simulink model "cx06_MA"  (Simulink 7.5)
settings: Solver=FixedStepDiscrete  StartTime=0.0  StopTime=10.0  RelTol=1e-3
undefined symbols (not defined in the file or in its folder): DiscIntNeverNeededParam, ECU555, int, motohawk_build_version, motohawk_trunc_name, motohawk_vardec_path
libraries: MotoHawk_lib x811, simulink x43, simulink_need_slupdate x1
(part 4 of 10)

== system cx06_MA/Outputs/Drive-by-Wire CAN Output ==
  Outputs : Inport  OutDataType=sfix(16)  OutScaling=2^0
  Bus Selector : BusSelector  OutputSignals=Hybrid.engine_Torque
  Constant : Constant  Value=0  OutDataType=sfix(16)  OutScaling=2^0
  Constant1 : Constant  Value=0  OutDataType=sfix(16)  OutScaling=2^0
  Data Type Conversion{,1..3} (4 alike) : DataTypeConversion  OutDataTypeMode=uint16  OutDataType=sfix(16)  OutScaling=2^0  OutDataTypeStr=uint16
  Gain1 : Gain  Gain=hex2dec('FFF')/5  ParameterDataType=sfix(16)  ParameterScaling=2^0  OutDataTypeMode=Specify via dialog  OutDataType=sint(16)  OutDataTypeStr=sint(16)
  Gain2 : Gain  Gain=hex2dec('FFF')/5  ParameterDataType=sfix(16)  ParameterScaling=2^0  OutDataTypeMode=Specify via dialog  OutDataType=sint(16)  OutDataTypeStr=sint(16)
  Product : Product  OutDataType=sfix(16)  OutScaling=2^0  RndMeth=Zero
  Product1 : Product  OutDataType=sfix(16)  OutScaling=2^0  RndMeth=Zero
  Send CAN Messages : MotoHawk_lib/CAN Blocks/Send CAN Messages  bus=-2  nam=['CAN_' num2str(1)]  msgl=CANTx_AO_169  pace=5  labelwires=on
  Subsystem : Subsystem
  Sum : Sum  Inputs=-+  OutDataType=sfix(16)  OutScaling=2^0
  Sum1 : Sum  Inputs=++|  OutDataType=sfix(16)  OutScaling=2^0
  Sum2 : Sum  Inputs=-+  OutDataType=sfix(16)  OutScaling=2^0
  Sum3 : Sum  Inputs=++|  OutDataType=sfix(16)  OutScaling=2^0
  motohawk_calibration : MotoHawk_lib/Calibration & Probing Blocks/motohawk_calibration  nam='Out1_Zero'  val=1  storage=Calibration  show_more=on  name_source=Use Parameter  data_type=Inherit from 'Default Value'  read_level=1  write_level=1  ovr_cals=on  view_as=Number  enum_struct={'Disabled', 'Enabled'}  vector_style=Wide Row  use_help_units=on  help='Output 0% Voltage'  units='V'  use_header_enum=off  row_header_enum={}  col_header_enum={}  use_min_max=off  min_val=0  max_val=5  use_precision=on  precision='1.3'  gain=1  offset=0  exp=1  use_mototune_group=off  mototune_group=motohawk_vardec_path(gcb)
  motohawk_calibration1 : MotoHawk_lib/Calibration & Probing Blocks/motohawk_calibration  nam='Out1_Full'  val=3.55  storage=Calibration  show_more=on  name_source=Use Parameter  data_type=Inherit from 'Default Value'  read_level=1  write_level=1  ovr_cals=on  view_as=Number  enum_struct={'Disabled', 'Enabled'}  vector_style=Wide Row  use_help_units=on  help='Output 100% Voltage'  units='V'  use_header_enum=off  row_header_enum={}  col_header_enum={}  use_min_max=off  min_val=0  max_val=5  use_precision=on  precision='1.3'  gain=1  offset=0  exp=1  use_mototune_group=off  mototune_group=motohawk_vardec_path(gcb)
  motohawk_calibration2 : MotoHawk_lib/Calibration & Probing Blocks/motohawk_calibration  nam='Out2_Zero'  val=0.5  storage=Calibration  show_more=on  name_source=Use Parameter  data_type=Inherit from 'Default Value'  read_level=1  write_level=1  ovr_cals=on  view_as=Number  enum_struct={'Disabled', 'Enabled'}  vector_style=Wide Row  use_help_units=on  help='Output1 0 Voltage'  units='V'  use_header_enum=off  row_header_enum={}  col_header_enum={}  use_min_max=off  min_val=0  max_val=5  use_precision=on  precision='1.3'  gain=1  offset=0  exp=1  use_mototune_group=off  mototune_group=motohawk_vardec_path(gcb)
  motohawk_calibration3 : MotoHawk_lib/Calibration & Probing Blocks/motohawk_calibration  nam='Out2_Full'  val=1.750  storage=Calibration  show_more=on  name_source=Use Parameter  data_type=Inherit from 'Default Value'  read_level=1  write_level=1  ovr_cals=on  view_as=Number  enum_struct={'Disabled', 'Enabled'}  vector_style=Wide Row  use_help_units=on  help='Output 100% Voltage'  units='V'  use_header_enum=off  row_header_enum={}  col_header_enum={}  use_min_max=off  min_val=0  max_val=5  use_precision=on  precision='1.3'  gain=1  offset=0  exp=1  use_mototune_group=off  mototune_group=motohawk_vardec_path(gcb)
  motohawk_override_abs{,1..3} (4 alike) : MotoHawk_lib/Calibration & Probing Blocks/motohawk_override_abs  SystemSampleTime=-1  parent_name='Override_Absolute'  parent_val=0  show_more=on  name_source=Use Output Wire Name  parent_read_level=1  parent_override_level=1  view_as=Number  enum_struct={'Disabled', 'Enabled'}  use_help_units=off  parent_help=''  parent_units=''  use_min_max=off  parent_min=-inf  parent_max=inf  use_precision=off  parent_precision=''  parent_gain=1  parent_offset=0  parent_exp=1  use_mototune_group=off  parent_group=motohawk_vardec_path(gcb)
  motohawk_probe{,1..3} (4 alike) : MotoHawk_lib/Calibration & Probing Blocks/motohawk_probe  nam='Probe'  show_more=on  name_source=Use Input Wire Name  read_level=1  view_as=Number  enum_struct={'Disabled', 'Enabled'}  vector_style=Wide Row  use_help_units=off  help=''  units=''  use_header_enum=off  row_header_enum={}  col_header_enum={}  use_precision=off  precision=''  gain=1  offset=0  exp=1  use_mototune_group=off  mototune_group=motohawk_vardec_path(gcb)
  motohawk_probe4 : MotoHawk_lib/Calibration & Probing Blocks/motohawk_probe  nam='AO_Checksum'  show_more=on  name_source=Use Parameter  read_level=1  view_as=Number  enum_struct={'Disabled', 'Enabled'}  vector_style=Wide Row  use_help_units=off  help=''  units=''  use_header_enum=off  row_header_enum={}  col_header_enum={}  use_precision=off  precision=''  gain=1  offset=0  exp=1  use_mototune_group=off  mototune_group=motohawk_vardec_path(gcb)
  wires:
  motohawk_override_abs/1 -> motohawk_probe1/1, Data Type Conversion2/1  "Reset_AO1"
  motohawk_override_abs1/1 -> motohawk_probe/1, Gain2/1  "Output_1"
  motohawk_override_abs2/1 -> motohawk_probe2/1, Data Type Conversion3/1  "Reset_AO2"
  motohawk_override_abs3/1 -> motohawk_probe3/1, Gain1/1  "Output_2"
  Constant/1 -> motohawk_override_abs/1  "Reset_AO1"
  Constant1/1 -> motohawk_override_abs2/1  "Reset_AO2"
  Sum/1 -> Product/1
  motohawk_calibration/1 -> Sum/1, Sum1/1
  motohawk_calibration1/1 -> Sum/2
  Product/1 -> Sum1/2
  Sum1/1 -> motohawk_override_abs1/1  "Output_1"
  Sum2/1 -> Product1/1
  motohawk_calibration2/1 -> Sum3/1, Sum2/1
  motohawk_calibration3/1 -> Sum2/2
  Product1/1 -> Sum3/2
  Sum3/1 -> motohawk_override_abs3/1  "Output_2"
  Outputs/1 -> Bus Selector/1
  Bus Selector/1 -> Product/2, Product1/2  "<engine_Torque>"
  Subsystem/1(Checksum) -> Send CAN Messages/5, motohawk_probe4/1  "Parity"
  Gain1/1 -> Data Type Conversion1/1  "Output_2"
  Gain2/1 -> Data Type Conversion/1  "Output_1"
  Data Type Conversion/1 -> Send CAN Messages/2, Subsystem/2(Output1)  "Output_1"
  Data Type Conversion1/1 -> Send CAN Messages/4, Subsystem/4(Output2)  "Output_2"
  Data Type Conversion2/1 -> Send CAN Messages/1, Subsystem/1(Reset_AO1)  "Reset_AO1"
  Data Type Conversion3/1 -> Send CAN Messages/3, Subsystem/3(Reset_AO2)  "Reset_AO2"

== system cx06_MA/Outputs/Fiat CAN Output ==
  note: NOTE:
      | Message $2F0
      | allows ECU to do
      | "supervisory checking"
      | on ABS
  Inputs : Inport  OutDataType=sfix(16)  OutScaling=2^0
  Bus Selector1 : BusSelector  OutputSignals=GMLAN.FL_Whl_Spd,GMLAN.FR_Whl_Spd,GMLAN.RL_Whl_Spd,GMLAN.RR_Whl_Spd
  Constant : Constant  OutDataType=sfix(16)  OutScaling=2^0
  Constant1 : Constant  Value=0  OutDataType=sfix(16)  OutScaling=2^0
  MinMax{,1..3} (4 alike) : MinMax  Function=max  Inputs=2  OutDataType=sfix(16)  OutScaling=2^0
  Send CAN Messages : MotoHawk_lib/CAN Blocks/Send CAN Messages  bus=-2  nam=['CAN_' num2str(1)]  msgl=CANTx_FIAT_280  pace=2  labelwires=on
  Send CAN Messages1 : MotoHawk_lib/CAN Blocks/Send CAN Messages  bus=-2  nam=['CAN_' num2str(1)]  msgl=CANTx_FIAT_2F0  pace=2  labelwires=on
  motohawk_calibration : MotoHawk_lib/Calibration & Probing Blocks/motohawk_calibration  nam='Wheel_Speed_Validities'  val=0  storage=Calibration  show_more=on  name_source=Use Parameter  data_type=uint8  read_level=1  write_level=1  ovr_cals=on  view_as=Enumeration  enum_struct={'Valid', 'Invalid'}  vector_style=Wide Row  use_help_units=on  help='Sets Validity bit for each wheels output on CAN'  units=''  use_header_enum=off  row_header_enum={}  col_header_enum={}  use_min_max=off  min_val=-inf  max_val=inf  use_precision=off  precision=''  gain=1  offset=0  exp=1  use_mototune_group=off  mototune_group=motohawk_vardec_path(gcb)
  motohawk_calibration1 : MotoHawk_lib/Calibration & Probing Blocks/motohawk_calibration  nam='Min_Wheel_Vel'  val=0  storage=Calibration  show_more=on  name_source=Use Parameter  data_type=double  read_level=1  write_level=1  ovr_cals=on  view_as=Number  enum_struct={'Valid', 'Invalid'}  vector_style=Wide Row  use_help_units=on  help='prevents ECU derating in first gear'  units=''  use_header_enum=off  row_header_enum={}  col_header_enum={}  use_min_max=off  min_val=-inf  max_val=inf  use_precision=on  precision='3.1'  gain=1  offset=0  exp=1  use_mototune_group=off  mototune_group=motohawk_vardec_path(gcb)
  motohawk_override_abs{,1..7} (8 alike) : MotoHawk_lib/Calibration & Probing Blocks/motohawk_override_abs  SystemSampleTime=-1  parent_name='Override_Absolute'  parent_val=0  show_more=on  name_source=Use Output Wire Name  parent_read_level=1  parent_override_level=1  view_as=Number  enum_struct={'Disabled', 'Enabled'}  use_help_units=off  parent_help=''  parent_units=''  use_min_max=off  parent_min=-inf  parent_max=inf  use_precision=off  parent_precision=''  parent_gain=1  parent_offset=0  parent_exp=1  use_mototune_group=off  parent_group=motohawk_vardec_path(gcb)
  motohawk_probe{,1..7} (8 alike) : MotoHawk_lib/Calibration & Probing Blocks/motohawk_probe  nam='Probe'  show_more=on  name_source=Use Input Wire Name  read_level=1  view_as=Number  enum_struct={'Disabled', 'Enabled'}  vector_style=Wide Row  use_help_units=off  help=''  units=''  use_header_enum=off  row_header_enum={}  col_header_enum={}  use_precision=off  precision=''  gain=1  offset=0  exp=1  use_mototune_group=off  mototune_group=motohawk_vardec_path(gcb)
  wires:
  Inputs/1 -> Bus Selector1/1
  motohawk_override_abs/1 -> Send CAN Messages/1, motohawk_probe/1  "Wheel_Ang_Vel_FL_V"
  motohawk_override_abs1/1 -> Send CAN Messages/2, motohawk_probe1/1  "Wheel_Ang_Vel_FL"
  motohawk_override_abs2/1 -> Send CAN Messages/3, motohawk_probe2/1  "Wheel_Ang_Vel_FR_V"
  motohawk_override_abs3/1 -> Send CAN Messages/4, motohawk_probe3/1  "Wheel_Ang_Vel_FR"
  motohawk_override_abs4/1 -> Send CAN Messages/5, motohawk_probe4/1  "Wheel_Ang_Vel_RL_V"
  motohawk_override_abs5/1 -> Send CAN Messages/6, motohawk_probe5/1  "Wheel_Ang_Vel_RL"
  motohawk_override_abs6/1 -> Send CAN Messages/7, motohawk_probe6/1  "Wheel_Ang_Vel_RR_V"
  motohawk_override_abs7/1 -> Send CAN Messages/8, motohawk_probe7/1  "Wheel_Ang_Vel_RR"
  motohawk_calibration/1 -> motohawk_override_abs/1, motohawk_override_abs2/1, motohawk_override_abs4/1, motohawk_override_abs6/1  "Wheel_Ang_Vel_RR_V"
  Constant1/1 -> Send CAN Messages1/1, Send CAN Messages1/4, Send CAN Messages1/5, Send CAN Messages1/6, Send CAN Messages1/7, Send CAN Messages1/8, Send CAN Messages1/9, Send CAN Messages1/11, Send CAN Messages1/12, Send CAN Messages1/19, Send CAN Messages1/20, Send CAN Messages1/21, Send CAN Messages1/23, Send CAN Messages1/24, Send CAN Messages1/26, Send CAN Messages1/25, Send CAN Messages1/18, Send CAN Messages1/17, Send CAN Messages1/16, Send CAN Messages1/15, Send CAN Messages1/14, Send CAN Messages1/13, Send CAN Messages1/10  "Drv_Off_Assist_Status"
  Constant/1 -> Send CAN Messages1/2, Send CAN Messages1/3, Send CAN Messages1/22  "Brk_Pres_Sensor_Diag_Complete"
  MinMax/1 -> motohawk_override_abs1/1  "Wheel_Ang_Vel_FL"
  Bus Selector1/1 -> MinMax/1  "<FL_Whl_Spd>"
  MinMax1/1 -> motohawk_override_abs3/1  "Wheel_Ang_Vel_FR"
  Bus Selector1/2 -> MinMax1/1  "<FR_Whl_Spd>"
  motohawk_calibration1/1 -> MinMax1/2, MinMax/2, MinMax2/2, MinMax3/2
  MinMax2/1 -> motohawk_override_abs5/1  "Wheel_Ang_Vel_RL"
  Bus Selector1/3 -> MinMax2/1  "<RL_Whl_Spd>"
  Bus Selector1/4 -> MinMax3/1  "<RR_Whl_Spd>"
  MinMax3/1 -> motohawk_override_abs7/1  "Wheel_Ang_Vel_RR"

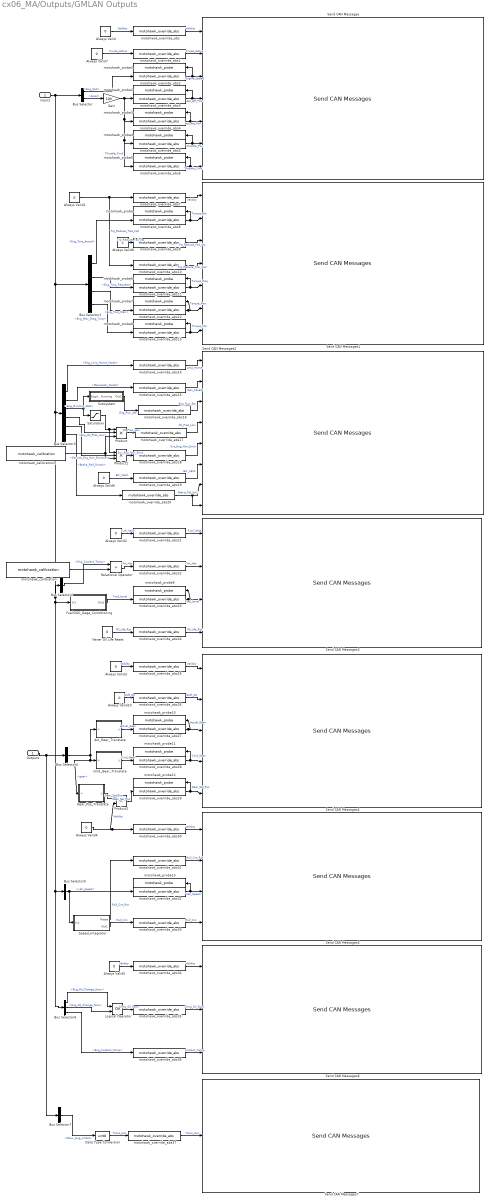
== system cx06_MA/Outputs/GMLAN Outputs ==
  Outputs : Inport  OutDataType=sfix(16)  OutScaling=2^0
  Inputs : Inport  Port=2  OutDataType=sfix(16)  OutScaling=2^0
  Act_Gear_Translate : Stateflow chart  TreatAsAtomicUnit=on
  Always Valid{,1..7,10} (9 alike) : Constant  Value=0  OutDataType=sfix(16)  OutScaling=2^0
  Always Valid8 : Constant  Value=2  OutDataType=sfix(16)  OutScaling=2^0
  Bus Selector : BusSelector  OutputSignals=Fiat.Engine Speed and Pedal Pos.Eng_Spd,Analog.Driver.Accel
  Bus Selector1 : BusSelector  OutputSignals=Fiat.Engine Torque.Eng_Torq_Actual,Fiat.Engine Torque.Eng_Torq_Request,Fiat.Engine Torque.Eng_Torq_Max,Fiat.Engine Torque.Eng_Max_Drag_Torq
  Bus Selector2 : BusSelector  OutputSignals=Fiat.Engine Temp.Eng_Coolant_Temp
  Bus Selector3 : BusSelector  OutputSignals="Fiat.Engine  General Status.Eng_Limp_Home_Mode,Fiat.Engine  General Status.Generator_Failed,Fiat.Engine  General Status.Eng_Running_Stat,Fiat.Engine  General Status.Eng_Oil_Pres_Low,Fiat.Engine  General Status.Service_Eng_Non_Emission,Fiat.Engine  General Status.Brake_Ped_Switch"
  Bus Selector4 : BusSelector  OutputSignals=Fiat/GMLAN.gear
  Bus Selector5 : BusSelector  OutputSignals=IPT.Status 2.veh_speed
  Bus Selector6 : BusSelector  OutputSignals="Fiat.Engine  General Status.Eng_Oil_Change_Soon,Fiat.Engine  General Status.Eng_Oil_Change_Now,Fiat.Engine Temp.Eng_Coolant_Temp"
  Bus Selector7 : BusSelector  OutputSignals=Hybrid.ESS_Outputs.Glow_plug_inhibit
  Cmd_Gear_Translate : Stateflow chart  TreatAsAtomicUnit=on
  Data Type Conversion : DataTypeConversion  OutDataTypeMode=uint8  OutDataType=sfix(16)  OutScaling=2^0  OutDataTypeStr=uint8
  Fuel/SOC_Gage_Conditioning : Subsystem
  Gain : Gain  Gain=100  ParameterDataType=sfix(16)  ParameterScaling=2^0  OutDataType=sfix(16)  OutScaling=2^0
  Gear_Pos_Translate : Stateflow chart  TreatAsAtomicUnit=on
  Logical Operator : Logic  Operator=OR  AllPortsSameDT=off  OutDataTypeMode=boolean  OutDataTypeStr=boolean
  Never Oil Life Reset : Constant  Value=0  OutDataType=sfix(16)  OutScaling=2^0
  Product : Product  Inputs=3  OutDataType=sfix(16)  OutScaling=2^0  RndMeth=Zero
  Product1 : Product  Inputs=3  OutDataType=sfix(16)  OutScaling=2^0  RndMeth=Zero
  Product2 : Product  OutDataType=sfix(16)  OutScaling=2^0  RndMeth=Zero
  Relational Operator : RelationalOperator  Operator=>  LogicOutDataTypeMode=boolean  OutDataTypeStr=boolean
  Saturation : Saturate  UpperLimit=1  LowerLimit=0
  Send CAN Messages : MotoHawk_lib/CAN Blocks/Send CAN Messages  bus=-2  nam=['CAN_' num2str(2)]  msgl=CANTx_GMLAN_110  pace=5  labelwires=on
  Send CAN Messages1 : MotoHawk_lib/CAN Blocks/Send CAN Messages  bus=-2  nam=['CAN_' num2str(2)]  msgl=CANTx_GMLAN_120  pace=5  labelwires=on
  Send CAN Messages2 : MotoHawk_lib/CAN Blocks/Send CAN Messages  bus=-2  nam=['CAN_' num2str(2)]  msgl=CANTx_GMLAN_300  pace=5  labelwires=on
  Send CAN Messages3 : MotoHawk_lib/CAN Blocks/Send CAN Messages  bus=-2  nam=['CAN_' num2str(2)]  msgl=CANTx_GMLAN_308  pace=5  labelwires=on
  Send CAN Messages4 : MotoHawk_lib/CAN Blocks/Send CAN Messages  bus=-2  nam=['CAN_' num2str(2)]  msgl=CANTx_GMLAN_320  pace=5  labelwires=on
  Send CAN Messages5 : MotoHawk_lib/CAN Blocks/Send CAN Messages  bus=-2  nam=['CAN_' num2str(2)]  msgl=CANTx_GMLAN_410  pace=5  labelwires=on
  Send CAN Messages6 : MotoHawk_lib/CAN Blocks/Send CAN Messages  bus=-2  nam=['CAN_' num2str(2)]  msgl=CANTx_GMLAN_510  pace=5  labelwires=on
  Send CAN Messages7 : MotoHawk_lib/CAN Blocks/Send CAN Messages  bus=-2  nam='CAN_2'  msgl=CANTx_GMLAN_520  pace=5  labelwires=on
  Speed_Integrator : Subsystem
  Subsystem : Subsystem
  motohawk_calibration : MotoHawk_lib/Calibration & Probing Blocks/motohawk_calibration  nam='Coolant_Temp_Warning_Thres'  val=115  storage=Calibration  show_more=off  name_source=Use Parameter  data_type=Inherit from 'Default Value'  read_level=1  write_level=1  ovr_cals=on  view_as=Number  enum_struct={'Disabled', 'Enabled'}  vector_style=Wide Row  use_help_units=off  help=''  units=''  use_header_enum=off  row_header_enum={}  col_header_enum={}  use_min_max=off  min_val=-inf  max_val=inf  use_precision=off  precision=''  gain=1  offset=0  exp=1  use_mototune_group=off  mototune_group=motohawk_vardec_path(gcb)
  motohawk_calibration1 : MotoHawk_lib/Calibration & Probing Blocks/motohawk_calibration  nam='CheckEngineLights'  val=1  storage=Calibration  show_more=on  name_source=Use Parameter  data_type=uint8  read_level=1  write_level=1  ovr_cals=on  view_as=Enumeration  enum_struct={'Disabled', 'Enabled'}  vector_style=Wide Row  use_help_units=off  help=''  units=''  use_header_enum=off  row_header_enum={}  col_header_enum={}  use_min_max=off  min_val=-inf  max_val=inf  use_precision=off  precision=''  gain=1  offset=0  exp=1  use_mototune_group=off  mototune_group=motohawk_vardec_path(gcb)
  motohawk_override_abs : MotoHawk_lib/Calibration & Probing Blocks/motohawk_override_abs  SystemSampleTime=-1  parent_name='Validity_110'  parent_val=0  show_more=on  name_source=Use Parameter  parent_read_level=1  parent_override_level=1  view_as=Number  enum_struct={'Disabled', 'Enabled'}  use_help_units=off  parent_help=''  parent_units=''  use_min_max=off  parent_min=-inf  parent_max=inf  use_precision=off  parent_precision=''  parent_gain=1  parent_offset=0  parent_exp=1  use_mototune_group=off  parent_group=motohawk_vardec_path(gcb)
  motohawk_override_abs{1..6,8..18,20,22..24,26..29,31..33,35..37} (31 alike) : MotoHawk_lib/Calibration & Probing Blocks/motohawk_override_abs  SystemSampleTime=-1  parent_name='Override_Absolute'  parent_val=0  show_more=on  name_source=Use Output Wire Name  parent_read_level=1  parent_override_level=1  view_as=Number  enum_struct={'Disabled', 'Enabled'}  use_help_units=off  parent_help=''  parent_units=''  use_min_max=off  parent_min=-inf  parent_max=inf  use_precision=off  parent_precision=''  parent_gain=1  parent_offset=0  parent_exp=1  use_mototune_group=off  parent_group=motohawk_vardec_path(gcb)
  motohawk_override_abs19 : MotoHawk_lib/Calibration & Probing Blocks/motohawk_override_abs  SystemSampleTime=-1  parent_name='Validity_300'  parent_val=0  show_more=on  name_source=Use Parameter  parent_read_level=1  parent_override_level=1  view_as=Number  enum_struct={'Disabled', 'Enabled'}  use_help_units=off  parent_help=''  parent_units=''  use_min_max=off  parent_min=-inf  parent_max=inf  use_precision=off  parent_precision=''  parent_gain=1  parent_offset=0  parent_exp=1  use_mototune_group=off  parent_group=motohawk_vardec_path(gcb)
  motohawk_override_abs21 : MotoHawk_lib/Calibration & Probing Blocks/motohawk_override_abs  SystemSampleTime=-1  parent_name='Validity_308'  parent_val=0  show_more=on  name_source=Use Parameter  parent_read_level=1  parent_override_level=1  view_as=Number  enum_struct={'Disabled', 'Enabled'}  use_help_units=off  parent_help=''  parent_units=''  use_min_max=off  parent_min=-inf  parent_max=inf  use_precision=off  parent_precision=''  parent_gain=1  parent_offset=0  parent_exp=1  use_mototune_group=off  parent_group=motohawk_vardec_path(gcb)
  motohawk_override_abs25 : MotoHawk_lib/Calibration & Probing Blocks/motohawk_override_abs  SystemSampleTime=-1  parent_name='Validity_320'  parent_val=0  show_more=on  name_source=Use Parameter  parent_read_level=1  parent_override_level=1  view_as=Number  enum_struct={'Disabled', 'Enabled'}  use_help_units=off  parent_help=''  parent_units=''  use_min_max=off  parent_min=-inf  parent_max=inf  use_precision=off  parent_precision=''  parent_gain=1  parent_offset=0  parent_exp=1  use_mototune_group=off  parent_group=motohawk_vardec_path(gcb)
  motohawk_override_abs30 : MotoHawk_lib/Calibration & Probing Blocks/motohawk_override_abs  SystemSampleTime=-1  parent_name='Validity_410'  parent_val=0  show_more=on  name_source=Use Parameter  parent_read_level=1  parent_override_level=1  view_as=Number  enum_struct={'Disabled', 'Enabled'}  use_help_units=off  parent_help=''  parent_units=''  use_min_max=off  parent_min=-inf  parent_max=inf  use_precision=off  parent_precision=''  parent_gain=1  parent_offset=0  parent_exp=1  use_mototune_group=off  parent_group=motohawk_vardec_path(gcb)
  motohawk_override_abs34 : MotoHawk_lib/Calibration & Probing Blocks/motohawk_override_abs  SystemSampleTime=-1  parent_name='Validity_510'  parent_val=0  show_more=on  name_source=Use Parameter  parent_read_level=1  parent_override_level=1  view_as=Number  enum_struct={'Disabled', 'Enabled'}  use_help_units=off  parent_help=''  parent_units=''  use_min_max=off  parent_min=-inf  parent_max=inf  use_precision=off  parent_precision=''  parent_gain=1  parent_offset=0  parent_exp=1  use_mototune_group=off  parent_group=motohawk_vardec_path(gcb)
  motohawk_override_abs7 : MotoHawk_lib/Calibration & Probing Blocks/motohawk_override_abs  SystemSampleTime=-1  parent_name='Validity_120'  parent_val=0  show_more=on  name_source=Use Parameter  parent_read_level=1  parent_override_level=1  view_as=Number  enum_struct={'Disabled', 'Enabled'}  use_help_units=off  parent_help=''  parent_units=''  use_min_max=off  parent_min=-inf  parent_max=inf  use_precision=off  parent_precision=''  parent_gain=1  parent_offset=0  parent_exp=1  use_mototune_group=off  parent_group=motohawk_vardec_path(gcb)
  motohawk_probe{,1..13} (14 alike) : MotoHawk_lib/Calibration & Probing Blocks/motohawk_probe  nam='Probe'  show_more=on  name_source=Use Input Wire Name  read_level=1  view_as=Number  enum_struct={'Disabled', 'Enabled'}  vector_style=Wide Row  use_help_units=off  help=''  units=''  use_header_enum=off  row_header_enum={}  col_header_enum={}  use_precision=off  precision=''  gain=1  offset=0  exp=1  use_mototune_group=off  mototune_group=motohawk_vardec_path(gcb)
  wires:
  motohawk_override_abs/1 -> Send CAN Messages/1  "Validity"
  motohawk_override_abs1/1 -> Send CAN Messages/2  "Cruise_Active"
  motohawk_override_abs2/1 -> Send CAN Messages/3, motohawk_probe1/1  "Engine_Speed"
  motohawk_override_abs3/1 -> Send CAN Messages/4, motohawk_probe2/1  "Acc_Eff_Pos"
  motohawk_override_abs4/1 -> Send CAN Messages/5, motohawk_probe3/1  "Acc_Act_Pos"
  motohawk_override_abs5/1 -> Send CAN Messages/6, motohawk_probe4/1  "Throttle_Pos"
  motohawk_override_abs6/1 -> Send CAN Messages/7, motohawk_probe5/1  "Throttle_Cmd"
  Always Valid/1 -> motohawk_override_abs/1  "Validity"
  Always Valid1/1 -> motohawk_override_abs7/1, motohawk_override_abs10/1  "Trq_Reduce_Trac_Fail"
  motohawk_override_abs7/1 -> Send CAN Messages1/1  "Validity"
  motohawk_override_abs8/1 -> Send CAN Messages1/2, motohawk_probe/1  "Torque_Act"
  motohawk_override_abs9/1 -> Send CAN Messages1/3  "Trq_Reduce_Fail_Sts"
  motohawk_override_abs10/1 -> Send CAN Messages1/4  "Trq_Reduce_Trac_Fail"
  motohawk_override_abs11/1 -> Send CAN Messages1/5, motohawk_probe6/1  "Torque_Req"
  motohawk_override_abs12/1 -> Send CAN Messages1/6, motohawk_probe7/1  "Torque_Max"
  motohawk_override_abs13/1 -> Send CAN Messages1/7, motohawk_probe8/1  "Torque_Min"
  motohawk_override_abs14/1 -> Send CAN Messages2/1  "Limp_Home"
  motohawk_override_abs15/1 -> Send CAN Messages2/2  "Gen_Failed"
  motohawk_override_abs16/1 -> Send CAN Messages2/3  "Eng_Run_Sts"
  motohawk_override_abs17/1 -> Send CAN Messages2/4  "Oil_Pres_Low"
  motohawk_override_abs18/1 -> Send CAN Messages2/5  "Svc_Eng_Non_Emis"
  motohawk_override_abs19/1 -> Send CAN Messages2/6  "Brk_Valid"
  motohawk_override_abs20/1 -> Send CAN Messages2/7, Send CAN Messages2/8  "Brake_Pdl_Sw2"
  Always Valid2/1 -> motohawk_override_abs21/1  "Fuel_Valid"
  motohawk_override_abs21/1 -> Send CAN Messages3/1  "Fuel_Valid"
  motohawk_override_abs22/1 -> Send CAN Messages3/2  "Clnt_Hot"
  motohawk_override_abs23/1 -> Send CAN Messages3/3, motohawk_probe9/1  "Fuel_Level"
  motohawk_override_abs24/1 -> Send CAN Messages3/4  "Oil_Life_Rst"
  motohawk_override_abs25/1 -> Send CAN Messages4/1  "Validity"
  motohawk_override_abs26/1 -> Send CAN Messages4/2  "Shift_Dir"
  motohawk_override_abs27/1 -> Send CAN Messages4/3, motohawk_probe10/1  "Actual_Gear"
  motohawk_override_abs28/1 -> Send CAN Messages4/4, motohawk_probe11/1  "Cmd_Gear"
  motohawk_override_abs29/1 -> Send CAN Messages4/5, motohawk_probe12/1  "Gear_Sel_Pos"
  Always Valid3/1 -> motohawk_override_abs25/1  "Validity"
  Always Valid4/1 -> motohawk_override_abs30/1, Product2/2  "Validity"
  motohawk_override_abs30/1 -> Send CAN Messages5/1  "Validity"
  motohawk_override_abs31/1 -> Send CAN Messages5/2  "Roll_Cnt_Rst"
  motohawk_override_abs32/1 -> Send CAN Messages5/3, motohawk_probe13/1  "Veh_Speed"
  motohawk_override_abs33/1 -> Send CAN Messages5/4  "Roll_Cnt"
  Always Valid5/1 -> motohawk_override_abs34/1  "Validity"
  motohawk_override_abs34/1 -> Send CAN Messages6/1  "Validity"
  motohawk_override_abs35/1 -> Send CAN Messages6/2  "Chng_Oil_Soon"
  motohawk_override_abs36/1 -> Send CAN Messages6/3  "Coolant_Temp"
  motohawk_override_abs37/1 -> Send CAN Messages7/1  "Trans_Hot"
  Always Valid6/1 -> motohawk_override_abs19/1  "Brk_Valid"
  Always Valid7/1 -> motohawk_override_abs1/1  "Cruise_Active"
  Inputs/1 -> Bus Selector/1, Bus Selector1/1, Bus Selector3/1, Bus Selector2/1, Bus Selector5/1, Bus Selector6/1, Fuel/SOC_Gage_Conditioning/1(In1)
  Bus Selector/1 -> motohawk_override_abs2/1  "<Eng_Spd>"
  Bus Selector/2 -> Gain/1  "<Accel>"
  Bus Selector1/1 -> motohawk_override_abs8/1  "<Eng_Torq_Actual>"
  Bus Selector1/2 -> motohawk_override_abs11/1  "<Eng_Torq_Request>"
  Bus Selector1/3 -> motohawk_override_abs12/1  "<Eng_Torq_Max>"
  Bus Selector1/4 -> motohawk_override_abs13/1  "<Eng_Max_Drag_Torq>"
  Always Valid8/1 -> motohawk_override_abs9/1  "Trq_Reduce_Fail_Sts"
  Always Valid10/1 -> motohawk_override_abs26/1  "Shift_Dir"
  Act_Gear_Translate/1(y) -> motohawk_override_abs27/1  "Actual_Gear"
  Cmd_Gear_Translate/1(y) -> motohawk_override_abs28/1  "Cmd_Gear"
  Outputs/1 -> Bus Selector4/1, Bus Selector7/1
  Bus Selector4/1 -> Act_Gear_Translate/1(u), Cmd_Gear_Translate/1(u), Gear_Pos_Translate/1(u)  "<gear>"
  Bus Selector5/1 -> motohawk_override_abs32/1, Speed_Integrator/1(In1)  "<veh_speed>"
  Subsystem/1(Out1) -> motohawk_override_abs16/1  "Eng_Run_Sts"
  Bus Selector6/3 -> motohawk_override_abs36/1  "<Eng_Coolant_Temp>"
  Bus Selector6/2 -> Logical Operator/2  "<Eng_Oil_Change_Now>"
  Bus Selector6/1 -> Logical Operator/1  "<Eng_Oil_Change_Soon>"
  Logical Operator/1 -> motohawk_override_abs35/1  "Chng_Oil_Soon"
  Speed_Integrator/1(Reset) -> motohawk_override_abs31/1  "Roll_Cnt_Rst"
  Speed_Integrator/2(Out1) -> motohawk_override_abs33/1  "Roll_Cnt"
  Never Oil Life Reset/1 -> motohawk_override_abs24/1  "Oil_Life_Rst"
  Bus Selector3/1 -> motohawk_override_abs14/1  "<Eng_Limp_Home_Mode>"
  Bus Selector3/2 -> motohawk_override_abs15/1  "<Generator_Failed>"
  Bus Selector3/3 -> Subsystem/1(Engine_Running), Saturation/1  "<Eng_Running_Stat>"
  Bus Selector3/6 -> motohawk_override_abs20/1  "<Brake_Ped_Switch>"
  Bus Selector2/1 -> Relational Operator/1  "<Eng_Coolant_Temp>"
  Relational Operator/1 -> motohawk_override_abs22/1  "Clnt_Hot"
  motohawk_calibration/1 -> Relational Operator/2
  Fuel/SOC_Gage_Conditioning/1(Out1) -> motohawk_override_abs23/1  "Fuel_Level"
  Bus Selector7/1 -> Data Type Conversion/1  "<Glow_plug_inhibit>"
  Data Type Conversion/1 -> motohawk_override_abs37/1  "Trans_Hot"
  Product/1 -> motohawk_override_abs17/1  "Oil_Pres_Low"
  Bus Selector3/4 -> Product/2  "<Eng_Oil_Pres_Low>"
  Saturation/1 -> Product/1, Product1/1
  Product1/1 -> motohawk_override_abs18/1  "Svc_Eng_Non_Emis"
  Bus Selector3/5 -> Product1/2  "<Service_Eng_Non_Emission>"
  Gear_Pos_Translate/1(y) -> Product2/1  "Gear_Sel_Pos"
  Product2/1 -> motohawk_override_abs29/1  "Gear_Sel_Pos"
  Gain/1 -> motohawk_override_abs3/1, motohawk_override_abs4/1, motohawk_override_abs5/1, motohawk_override_abs6/1  "Throttle_Cmd"
  motohawk_calibration1/1 -> Product/3, Product1/3

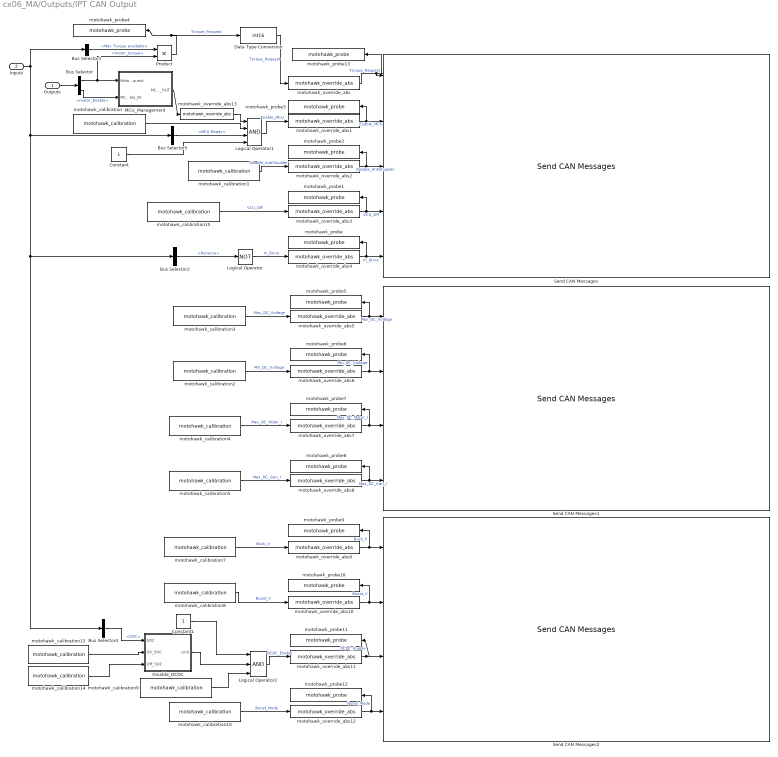
== system cx06_MA/Outputs/IPT CAN Output ==
  Outputs : Inport  OutDataType=sfix(16)  OutScaling=2^0
  Inputs : Inport  Port=2  OutDataType=sfix(16)  OutScaling=2^0
  Bus Selector : BusSelector  OutputSignals=Hybrid.motor_torque,Hybrid.motor_Enable
  Bus Selector1 : BusSelector  OutputSignals=IPT.Status 1.Max Torque available
  Bus Selector2 : BusSelector  OutputSignals=Analog.Trans.Reverse
  Bus Selector4 : BusSelector  OutputSignals=JCI.SOC
  Bus Selector5 : BusSelector  OutputSignals=IPT.Status 1.MCU Ready
  Constant : Constant  OutDataTypeMode=boolean  OutDataType=fixdt(1, 16)  OutScaling=2^0  OutDataTypeStr=boolean
  Constant1 : Constant  OutDataTypeMode=boolean  OutDataType=fixdt(1, 16)  OutScaling=2^0  OutDataTypeStr=boolean
  Data Type Conversion : DataTypeConversion  OutDataTypeMode=int16  OutDataType=sfix(16)  OutScaling=2^0  OutDataTypeStr=int16
  Disable_DCDC : Stateflow chart  TreatAsAtomicUnit=on
  Logical Operator : Logic  Operator=NOT  AllPortsSameDT=off  OutDataTypeMode=boolean  OutDataTypeStr=boolean
  Logical Operator1 : Logic  Inputs=4  AllPortsSameDT=off  OutDataTypeMode=boolean  OutDataTypeStr=boolean
  Logical Operator2 : Logic  Inputs=3  AllPortsSameDT=off  OutDataTypeMode=boolean  OutDataTypeStr=boolean
  MCU_Management : Subsystem
  Product : Product  OutDataType=sfix(16)  OutScaling=2^0  OutDataTypeStr=Inherit: Inherit via back propagation  RndMeth=Zero
  Send CAN Messages : MotoHawk_lib/CAN Blocks/Send CAN Messages  bus=-2  nam=['CAN_' num2str(1)]  msgl=CANTx_IPT_250  pace=5  labelwires=on
  Send CAN Messages1 : MotoHawk_lib/CAN Blocks/Send CAN Messages  bus=-2  nam=['CAN_' num2str(1)]  msgl=CANTx_IPT_318  pace=5  labelwires=on
  Send CAN Messages2 : MotoHawk_lib/CAN Blocks/Send CAN Messages  bus=-2  nam=['CAN_' num2str(1)]  msgl=CANTx_IPT_628  pace=5  labelwires=on
  motohawk_calibration : MotoHawk_lib/Calibration & Probing Blocks/motohawk_calibration  nam='Enable_IPT'  val=1  storage=Calibration  show_more=on  name_source=Use Parameter  data_type=uint8  read_level=1  write_level=1  ovr_cals=on  view_as=Enumeration  enum_struct={'Disabled', 'Enabled'}  vector_style=Wide Row  use_help_units=on  help='Enables the IPT Motor'  units=''  use_header_enum=off  row_header_enum={}  col_header_enum={}  use_min_max=off  min_val=-inf  max_val=inf  use_precision=off  precision=''  gain=1  offset=0  exp=1  use_mototune_group=off  mototune_group=motohawk_vardec_path(gcb)
  motohawk_calibration1 : MotoHawk_lib/Calibration & Probing Blocks/motohawk_calibration  nam='DisableAntiShudder'  val=0  storage=Calibration  show_more=on  name_source=Use Parameter  data_type=uint8  read_level=1  write_level=1  ovr_cals=on  view_as=Enumeration  enum_struct={'False', 'True'}  vector_style=Wide Row  use_help_units=on  help='This should really be run by the ABS'  units=''  use_header_enum=off  row_header_enum={}  col_header_enum={}  use_min_max=off  min_val=-inf  max_val=inf  use_precision=off  precision=''  gain=1  offset=0  exp=1  use_mototune_group=off  mototune_group=motohawk_vardec_path(gcb)
  motohawk_calibration10 : MotoHawk_lib/Calibration & Probing Blocks/motohawk_calibration  nam='DCDC_Mode'  val=0  storage=Calibration  show_more=on  name_source=Use Parameter  data_type=uint8  read_level=1  write_level=1  ovr_cals=on  view_as=Enumeration  enum_struct={'Buck', 'Boost'}  vector_style=Wide Row  use_help_units=on  help='Enable DCDC Converter'  units=''  use_header_enum=off  row_header_enum={}  col_header_enum={}  use_min_max=on  min_val=0  max_val=400  use_precision=on  precision=''  gain=1  offset=0  exp=1  use_mototune_group=off  mototune_group=motohawk_vardec_path(gcb)
  motohawk_calibration13 : MotoHawk_lib/Calibration & Probing Blocks/motohawk_calibration  nam='SOC_On_DCDC'  val=20  storage=Calibration  show_more=on  name_source=Use Parameter  data_type=uint8  read_level=1  write_level=1  ovr_cals=off  view_as=Number  enum_struct={'Disabled', 'Enabled'}  vector_style=Wide Row  use_help_units=on  help='SOC threshold to Enable DCDC Converter'  units=''  use_header_enum=off  row_header_enum={}  col_header_enum={}  use_min_max=on  min_val=0  max_val=100  use_precision=on  precision=''  gain=1  offset=0  exp=1  use_mototune_group=off  mototune_group=motohawk_vardec_path(gcb)
  motohawk_calibration14 : MotoHawk_lib/Calibration & Probing Blocks/motohawk_calibration  nam='SOC_Off_DCDC'  val=15  storage=Calibration  show_more=on  name_source=Use Parameter  data_type=uint8  read_level=1  write_level=1  ovr_cals=off  view_as=Number  enum_struct={'Disabled', 'Enabled'}  vector_style=Wide Row  use_help_units=on  help='SOC threshold to Enable DCDC Converter'  units=''  use_header_enum=off  row_header_enum={}  col_header_enum={}  use_min_max=on  min_val=0  max_val=100  use_precision=on  precision=''  gain=1  offset=0  exp=1  use_mototune_group=off  mototune_group=motohawk_vardec_path(gcb)
  motohawk_calibration15 : MotoHawk_lib/Calibration & Probing Blocks/motohawk_calibration  nam='VCUOff'  val=0  storage=Calibration  show_more=on  name_source=Use Parameter  data_type=uint8  read_level=1  write_level=1  ovr_cals=on  view_as=Enumeration  enum_struct={'False', 'True'}  vector_style=Wide Row  use_help_units=on  help='This should really be run by the ABS'  units=''  use_header_enum=off  row_header_enum={}  col_header_enum={}  use_min_max=off  min_val=-inf  max_val=inf  use_precision=off  precision=''  gain=1  offset=0  exp=1  use_mototune_group=off  mototune_group=motohawk_vardec_path(gcb)
  motohawk_calibration2 : MotoHawk_lib/Calibration & Probing Blocks/motohawk_calibration  nam='Min_Voltage'  val=195  storage=Calibration  show_more=on  name_source=Use Parameter  data_type=uint16  read_level=1  write_level=1  ovr_cals=on  view_as=Number  enum_struct={'Battery', 'Calibration'}  vector_style=Wide Row  use_help_units=off  help='Upper Voltage Limit'  units='V'  use_header_enum=off  row_header_enum={}  col_header_enum={}  use_min_max=on  min_val=0  max_val=400  use_precision=off  precision=''  gain=1  offset=0  exp=1  use_mototune_group=off  mototune_group=motohawk_vardec_path(gcb)
  motohawk_calibration3 : MotoHawk_lib/Calibration & Probing Blocks/motohawk_calibration  nam='Max_Voltage'  val=288  storage=Calibration  show_more=on  name_source=Use Parameter  data_type=uint16  read_level=1  write_level=1  ovr_cals=on  view_as=Number  enum_struct={'Battery', 'Calibration'}  vector_style=Wide Row  use_help_units=off  help='Upper Voltage Limit'  units='V'  use_header_enum=off  row_header_enum={}  col_header_enum={}  use_min_max=on  min_val=0  max_val=400  use_precision=off  precision=''  gain=1  offset=0  exp=1  use_mototune_group=off  mototune_group=motohawk_vardec_path(gcb)
  motohawk_calibration4 : MotoHawk_lib/Calibration & Probing Blocks/motohawk_calibration  nam='Max_Current'  val=400  storage=Calibration  show_more=on  name_source=Use Parameter  data_type=uint16  read_level=1  write_level=1  ovr_cals=on  view_as=Number  enum_struct={'Battery', 'Calibration'}  vector_style=Wide Row  use_help_units=off  help='Upper Voltage Limit'  units='V'  use_header_enum=off  row_header_enum={}  col_header_enum={}  use_min_max=on  min_val=0  max_val=400  use_precision=off  precision=''  gain=1  offset=0  exp=1  use_mototune_group=off  mototune_group=motohawk_vardec_path(gcb)
  motohawk_calibration5 : MotoHawk_lib/Calibration & Probing Blocks/motohawk_calibration  nam='Regen_Current'  val=400  storage=Calibration  show_more=on  name_source=Use Parameter  data_type=uint16  read_level=1  write_level=1  ovr_cals=on  view_as=Number  enum_struct={'Battery', 'Calibration'}  vector_style=Wide Row  use_help_units=off  help='Upper Voltage Limit'  units='V'  use_header_enum=off  row_header_enum={}  col_header_enum={}  use_min_max=on  min_val=0  max_val=400  use_precision=off  precision=''  gain=1  offset=0  exp=1  use_mototune_group=off  mototune_group=motohawk_vardec_path(gcb)
  motohawk_calibration7 : MotoHawk_lib/Calibration & Probing Blocks/motohawk_calibration  nam='DCDC_Buck_V'  val=14  storage=Calibration  show_more=on  name_source=Use Parameter  data_type=Inherit from 'Default Value'  read_level=1  write_level=1  ovr_cals=on  view_as=Number  enum_struct={'Disabled', 'Enabled'}  vector_style=Wide Row  use_help_units=on  help='Buck Converter Output V'  units='V'  use_header_enum=off  row_header_enum={}  col_header_enum={}  use_min_max=on  min_val=0  max_val=15  use_precision=on  precision='2.1'  gain=1  offset=0  exp=1  use_mototune_group=off  mototune_group=motohawk_vardec_path(gcb)
  motohawk_calibration8 : MotoHawk_lib/Calibration & Probing Blocks/motohawk_calibration  nam='DCDC_Boost_V'  val=0  storage=Calibration  show_more=on  name_source=Use Parameter  data_type=uint16  read_level=1  write_level=1  ovr_cals=on  view_as=Number  enum_struct={'Disabled', 'Enabled'}  vector_style=Wide Row  use_help_units=on  help='Boost Converter Output V'  units='V'  use_header_enum=off  row_header_enum={}  col_header_enum={}  use_min_max=on  min_val=0  max_val=400  use_precision=on  precision=''  gain=1  offset=0  exp=1  use_mototune_group=off  mototune_group=motohawk_vardec_path(gcb)
  motohawk_calibration9 : MotoHawk_lib/Calibration & Probing Blocks/motohawk_calibration  nam='DCDC_En'  val=1  storage=Calibration  show_more=on  name_source=Use Parameter  data_type=uint8  read_level=1  write_level=1  ovr_cals=on  view_as=Enumeration  enum_struct={'Disabled', 'Enabled'}  vector_style=Wide Row  use_help_units=on  help='Enable DCDC Converter'  units=''  use_header_enum=off  row_header_enum={}  col_header_enum={}  use_min_max=on  min_val=0  max_val=400  use_precision=on  precision=''  gain=1  offset=0  exp=1  use_mototune_group=off  mototune_group=motohawk_vardec_path(gcb)
  motohawk_override_abs : MotoHawk_lib/Calibration & Probing Blocks/motohawk_override_abs  SystemSampleTime=-1  parent_name='Filt_Torque_Request'  parent_val=0  show_more=on  name_source=Use Parameter  parent_read_level=1  parent_override_level=1  view_as=Number  enum_struct={'Disabled', 'Enabled'}  use_help_units=off  parent_help=''  parent_units=''  use_min_max=off  parent_min=-inf  parent_max=inf  use_precision=off  parent_precision=''  parent_gain=1  parent_offset=0  parent_exp=1  use_mototune_group=off  parent_group=motohawk_vardec_path(gcb)
  motohawk_override_abs{1..12} (12 alike) : MotoHawk_lib/Calibration & Probing Blocks/motohawk_override_abs  SystemSampleTime=-1  parent_name='Override_Absolute'  parent_val=0  show_more=on  name_source=Use Output Wire Name  parent_read_level=1  parent_override_level=1  view_as=Number  enum_struct={'Disabled', 'Enabled'}  use_help_units=off  parent_help=''  parent_units=''  use_min_max=off  parent_min=-inf  parent_max=inf  use_precision=off  parent_precision=''  parent_gain=1  parent_offset=0  parent_exp=1  use_mototune_group=off  parent_group=motohawk_vardec_path(gcb)
  motohawk_override_abs13 : MotoHawk_lib/Calibration & Probing Blocks/motohawk_override_abs  SystemSampleTime=-1  parent_name='motor_Enable'  parent_val=0  show_more=on  name_source=Use Parameter  parent_read_level=1  parent_override_level=1  view_as=Number  enum_struct={'Disabled', 'Enabled'}  use_help_units=off  parent_help=''  parent_units=''  use_min_max=off  parent_min=-inf  parent_max=inf  use_precision=off  parent_precision=''  parent_gain=1  parent_offset=0  parent_exp=1  use_mototune_group=off  parent_group=motohawk_vardec_path(gcb)
  motohawk_probe{,1..12} (13 alike) : MotoHawk_lib/Calibration & Probing Blocks/motohawk_probe  nam='Probe'  show_more=on  name_source=Use Input Wire Name  read_level=1  view_as=Number  enum_struct={'Disabled', 'Enabled'}  vector_style=Wide Row  use_help_units=off  help=''  units=''  use_header_enum=off  row_header_enum={}  col_header_enum={}  use_precision=off  precision=''  gain=1  offset=0  exp=1  use_mototune_group=off  mototune_group=motohawk_vardec_path(gcb)
  motohawk_probe13 : MotoHawk_lib/Calibration & Probing Blocks/motohawk_probe  nam='Filt_Torque_Request'  show_more=off  name_source=Use Parameter  read_level=1  view_as=Number  enum_struct={'Disabled', 'Enabled'}  vector_style=Wide Row  use_help_units=off  help=''  units=''  use_header_enum=off  row_header_enum={}  col_header_enum={}  use_precision=off  precision=''  gain=1  offset=0  exp=1  use_mototune_group=off  mototune_group=motohawk_vardec_path(gcb)
  wires:
  motohawk_override_abs/1 -> Send CAN Messages/1, motohawk_probe13/1  "Torque_Request"
  motohawk_override_abs1/1 -> Send CAN Messages/2, motohawk_probe3/1  "Enable_MCU"
  motohawk_override_abs2/1 -> Send CAN Messages/3, motohawk_probe2/1  "Disable_AntiShudder"
  motohawk_override_abs3/1 -> Send CAN Messages/4, motohawk_probe1/1  "VCU_Off"
  motohawk_override_abs4/1 -> Send CAN Messages/5, motohawk_probe/1  "In_Drive"
  motohawk_override_abs5/1 -> Send CAN Messages1/1, motohawk_probe5/1  "Max_DC_Voltage"
  motohawk_override_abs6/1 -> Send CAN Messages1/2, motohawk_probe6/1  "Min_DC_Voltage"
  motohawk_override_abs7/1 -> Send CAN Messages1/3, motohawk_probe7/1  "Max_DC_Motor_I"
  motohawk_override_abs8/1 -> Send CAN Messages1/4, motohawk_probe8/1  "Max_DC_Gen_I"
  motohawk_override_abs9/1 -> Send CAN Messages2/1, motohawk_probe9/1  "Buck_V"
  motohawk_override_abs10/1 -> Send CAN Messages2/2, motohawk_probe10/1  "Boost_V"
  motohawk_override_abs11/1 -> Send CAN Messages2/3, motohawk_probe11/1  "DCDC_Enable"
  motohawk_override_abs12/1 -> Send CAN Messages2/4, motohawk_probe12/1  "Boost_Mode"
  Outputs/1 -> Bus Selector/1
  Inputs/1 -> Bus Selector1/1, Bus Selector2/1, Bus Selector4/1, Bus Selector5/1
  Product/1 -> motohawk_probe4/1, Data Type Conversion/1  "Torque_Request"
  motohawk_calibration15/1 -> motohawk_override_abs3/1  "VCU_Off"
  motohawk_calibration1/1 -> motohawk_override_abs2/1  "Disable_AntiShudder"
  Bus Selector2/1 -> Logical Operator/1  "<Reverse>"
  Logical Operator/1 -> motohawk_override_abs4/1  "In_Drive"
  motohawk_calibration/1 -> Logical Operator1/2
  Logical Operator1/1 -> motohawk_override_abs1/1  "Enable_MCU"
  motohawk_calibration8/1 -> motohawk_override_abs10/1  "Boost_V"
  motohawk_calibration7/1 -> motohawk_override_abs9/1  "Buck_V"
  motohawk_calibration10/1 -> motohawk_override_abs12/1  "Boost_Mode"
  Logical Operator2/1 -> motohawk_override_abs11/1  "DCDC_Enable"
  Bus Selector1/1 -> Product/1  "<Max Torque available>"
  Data Type Conversion/1 -> motohawk_override_abs/1  "Torque_Request"
  Bus Selector/1 -> Product/2, MCU_Management/1(Motor_Torque_Request)  "<motor_torque>"
  motohawk_override_abs13/1 -> Logical Operator1/1
  MCU_Management/1(MCU_Enable_OUT) -> motohawk_override_abs13/1
  Bus Selector/2 -> MCU_Management/2(MCU_Enable_IN)  "<motor_Enable>"
  motohawk_calibration13/1 -> Disable_DCDC/2(On_SOC)
  motohawk_calibration14/1 -> Disable_DCDC/3(Off_SOC)
  Bus Selector5/1 -> Logical Operator1/3  "<MCU Ready>"
  motohawk_calibration3/1 -> motohawk_override_abs5/1  "Max_DC_Voltage"
  motohawk_calibration2/1 -> motohawk_override_abs6/1  "Min_DC_Voltage"
  motohawk_calibration4/1 -> motohawk_override_abs7/1  "Max_DC_Motor_I"
  motohawk_calibration5/1 -> motohawk_override_abs8/1  "Max_DC_Gen_I"
  Bus Selector4/1 -> Disable_DCDC/1(SOC)  "<SOC>"
  Disable_DCDC/1(cmd) -> Logical Operator2/2
  motohawk_calibration9/1 -> Logical Operator2/3
  Constant/1 -> Logical Operator1/4
  Constant1/1 -> Logical Operator2/1

== system cx06_MA/Outputs/JCI CAN Output ==
  Constant : Constant  Value=hex2dec('00FF6B')  OutDataType=sfix(16)  OutScaling=2^0
  Constant{1,3..6} (5 alike) : Constant  Value=0  OutDataType=sfix(16)  OutScaling=2^0
  Constant2 : Constant  Value=20  OutDataType=sfix(16)  OutScaling=2^0
  Constant7 : Constant  OutDataTypeMode=boolean  OutDataType=fixdt(1, 16)  OutScaling=2^0  OutDataTypeStr=boolean
  Send CAN Messages : MotoHawk_lib/CAN Blocks/Send CAN Messages  bus=-2  nam=['CAN_' num2str(1)]  msgl=CANTx_JCI_460  pace=5  labelwires=on
  Send CAN Messages1 : MotoHawk_lib/CAN Blocks/Send CAN Messages  bus=-2  nam=['CAN_' num2str(1)]  msgl=CANTx_JCI_462  pace=5  labelwires=on
  motohawk_calibration : MotoHawk_lib/Calibration & Probing Blocks/motohawk_calibration  nam='ISO_Enable'  val=0  storage=Calibration  show_more=on  name_source=Use Parameter  data_type=uint8  read_level=1  write_level=1  ovr_cals=on  view_as=Enumeration  enum_struct={'Disabled', 'Enabled'}  vector_style=Wide Row  use_help_units=on  help='Enable Ground Fault Meter'  units=''  use_header_enum=off  row_header_enum={}  col_header_enum={}  use_min_max=off  min_val=-inf  max_val=inf  use_precision=off  precision=''  gain=1  offset=0  exp=1  use_mototune_group=off  mototune_group=motohawk_vardec_path(gcb)
  motohawk_override_abs{,1..9} (10 alike) : MotoHawk_lib/Calibration & Probing Blocks/motohawk_override_abs  SystemSampleTime=-1  parent_name='Override_Absolute'  parent_val=0  show_more=on  name_source=Use Output Wire Name  parent_read_level=1  parent_override_level=1  view_as=Number  enum_struct={'Disabled', 'Enabled'}  use_help_units=off  parent_help=''  parent_units=''  use_min_max=off  parent_min=-inf  parent_max=inf  use_precision=off  parent_precision=''  parent_gain=1  parent_offset=0  parent_exp=1  use_mototune_group=off  parent_group=motohawk_vardec_path(gcb)
  motohawk_probe{,1..8} (9 alike) : MotoHawk_lib/Calibration & Probing Blocks/motohawk_probe  nam='Probe'  show_more=on  name_source=Use Input Wire Name  read_level=1  view_as=Number  enum_struct={'Disabled', 'Enabled'}  vector_style=Wide Row  use_help_units=off  help=''  units=''  use_header_enum=off  row_header_enum={}  col_header_enum={}  use_precision=off  precision=''  gain=1  offset=0  exp=1  use_mototune_group=off  mototune_group=motohawk_vardec_path(gcb)
  wires:
  motohawk_override_abs/1 -> Send CAN Messages/1, motohawk_probe/1  "Contactor_Enable"
  motohawk_override_abs1/1 -> Send CAN Messages/2, motohawk_probe1/1  "Contactor_On"
  motohawk_override_abs2/1 -> Send CAN Messages/3, motohawk_probe2/1  "BMS_Standby"
  motohawk_override_abs3/1 -> Send CAN Messages/4, motohawk_probe3/1  "Charger_Ready"
  motohawk_override_abs4/1 -> Send CAN Messages/5, motohawk_probe4/1  "Emergency_Contactor_Off"
  motohawk_override_abs5/1 -> Send CAN Messages/6, motohawk_probe5/1  "Quit_Batt_Locked"
  motohawk_override_abs6/1 -> Send CAN Messages/7, motohawk_probe6/1  "Ambient_Temp"
  motohawk_override_abs7/1 -> Send CAN Messages/8, motohawk_probe7/1  "Air_Pres"
  motohawk_override_abs8/1 -> Send CAN Messages1/1  "Reguest_PGN"
  Constant/1 -> motohawk_override_abs8/1  "Reguest_PGN"
  motohawk_override_abs9/1 -> Send CAN Messages/9, motohawk_probe8/1  "ISO_On"
  Constant7/1 -> motohawk_override_abs1/1, motohawk_override_abs/1  "Contactor_On"
  motohawk_calibration/1 -> motohawk_override_abs9/1  "ISO_On"
  Constant6/1 -> motohawk_override_abs2/1  "BMS_Standby"
  Constant5/1 -> motohawk_override_abs3/1  "Charger_Ready"
  Constant4/1 -> motohawk_override_abs4/1  "Emergency_Contactor_Off"
  Constant3/1 -> motohawk_override_abs5/1  "Quit_Batt_Locked"
  Constant2/1 -> motohawk_override_abs6/1  "Ambient_Temp"
  Constant1/1 -> motohawk_override_abs7/1  "Air_Pres"
